simulink model "SUPERSONIC_ALTITUDEHOLD_AUTOPILOT_SIMULINK"  (R2020a)
settings: Solver=VariableStepAuto  StartTime=0.0  StopTime=150  RelTol=1e-3
values from neighbouring files (symbols this model uses):
  u0 = 1742    [SUPERSONIC_ALTITUDEHOLD_AUTOPILOT_MATLAB.m]
libraries: cstblocks x3, simulink x1
settings Model: Creator=AHSAN  LastModifiedBy=AHSAN

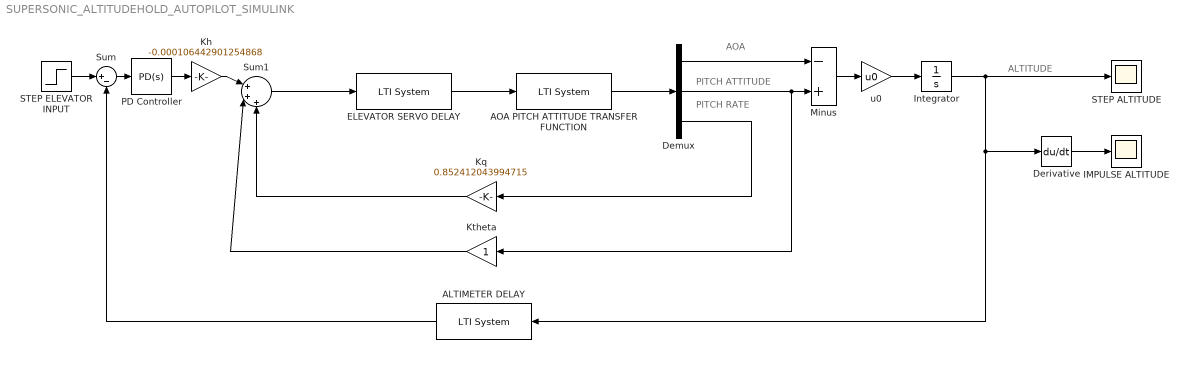
== system SUPERSONIC_ALTITUDEHOLD_AUTOPILOT_SIMULINK ==
  note: ALTITUDE
  note: PITCH RATE
  note: PITCH ATTITUDE
  note: AOA
  ALTIMETER DELAY : cstblocks/LTI System  sys=tf(1,[1 1])  IC=[]
  AOA PITCH ATTITUDE TRANSFER FUNCTION : cstblocks/LTI System  sys=SYSTEM  IC=[]
  Demux : Demux  Outputs=3
  Derivative : Derivative
  ELEVATOR SERVO DELAY : cstblocks/LTI System  sys=tf(10,[1 10])  IC=[]
  IMPULSE ALTITUDE : Scope
  Integrator : Integrator
  Kh : Gain  Gain=-0.000106442901254868
  Kq : Gain  Gain=0.852412043994715
  Ktheta : Gain
  Minus : Sum  Inputs=-+
  PD Controller : simulink/Continuous/PID Controller  Controller=PD  Form=Parallel  TimeDomain=Continuous-time  UseExternalTs=off  SampleTime=-1  IntegratorMethod=Forward Euler  FilterMethod=Forward Euler  ControllerParametersSource=internal  P=0.702446637657272  I=0  D=2.92686099023863  UseFilter=on  N=100  TunerSelectOption=Transfer Function Based (PID Tuner App)  InitialConditionSource=internal  InitialConditionForIntegrator=0  InitialConditionForFilter=0  DifferentiatorICPrevScaledInput=0  ExternalReset=none  TrackingMode=off  Kt=1  LimitOutput=off  UpperSaturationLimit=inf  LowerSaturationLimit=-inf  LinearizeAsGain=on  AntiWindupMode=none  Kb=1  POutMin=[]  POutMax=[]  IOutMin=[]  IOutMax=[]  DOutMin=[]  DOutMax=[]  NOutMin=[]  NOutMax=[]  SumOutMin=[]  SumOutMax=[]  SaturationOutMin=[]  SaturationOutMax=[]  PParamMin=[]  PParamMax=[]  IParamMin=[]  IParamMax=[]  DParamMin=[]  DParamMax=[]  NParamMin=[]  NParamMax=[]  KbParamMin=[]  KbParamMax=[]  KtParamMin=[]  KtParamMax=[]  KbOutMin=[]  KbOutMax=[]  KtOutMin=[]  KtOutMax=[]  IntegratorOutMin=[]  IntegratorOutMax=[]  FilterOutMin=[]  FilterOutMax=[]  SumI1OutMin=[]  SumI1OutMax=[]  SumI2OutMin=[]  SumI2OutMax=[]  SumI3OutMin=[]  SumI3OutMax=[]  SumI4OutMin=[]  SumI4OutMax=[]  SumDOutMin=[]  SumDOutMax=[]  DifferentiatorOutMin=[]  DifferentiatorOutMax=[]  FilterDiffOutCoefMin=[]  FilterDiffOutCoefMax=[]  ReciprocalOutMin=[]  ReciprocalOutMax=[]  SumDenOutMin=[]  SumDenOutMax=[]  SumNumOutMin=[]  SumNumOutMax=[]  DivideOutMin=[]  DivideOutMax=[]  UdiffTsProdOutMin=[]  UdiffTsProdOutMax=[]  NTsProdOutMin=[]  NTsProdOutMax=[]  UintegralTsProdOutMin=[]  UintegralTsProdOutMax=[]  UngainTsProdOutMin=[]  UngainTsProdOutMax=[]  IntegratorContinuousStateAttributes=''  IntegratorStateMustResolveToSignalObject=off  IntegratorRTWStateStorageClass=Auto  FilterContinuousStateAttributes=''  FilterStateMustResolveToSignalObject=off  FilterRTWStateStorageClass=Auto  ParallelPVariant=InternalParameters  IdealPVariant=Disabled  IVariant=Disabled  DVariant=InternalParameters  IntegratorVariant=Disabled  SatVariant=Disabled  AWVariant=Disabled  PCopyVariant=Disabled  TRVariant=Disabled  FdbkBlocksVariant=Forward  IdealPFdbkVariant=Disabled  SatFdbkVariant=Disabled  DerivativeFilterVariant=ContFilter  NVariant=InternalParameters  NCopyVariant=Disabled  FilterICVariant=InternalICsFilter  IntegratorICVariant=Disabled  ExternalResetVariant=Disabled  TRSumVariant=Passthrough  SumFdbkVariant=Disabled  SumVariant=Sum_PD  TsampFilterVariant=InternalTs  TsampNgainVariant=Passthrough  TsampIntegralVariant=Disabled_SignalSpec
  STEP ALTITUDE : Scope
  STEP ELEVATOR INPUT : Step  Time=0  SampleTime=0
  Sum : Sum  Inputs=|+-
  Sum1 : Sum  Inputs=|+++
  u0 : Gain  Gain=u0
  wires:
  ELEVATOR SERVO DELAY/1 -> AOA PITCH ATTITUDE TRANSFER FUNCTION/1
  AOA PITCH ATTITUDE TRANSFER FUNCTION/1 -> Demux/1
  Minus/1 -> u0/1
  u0/1 -> Integrator/1
  Integrator/1 -> STEP ALTITUDE/1, Derivative/1, ALTIMETER DELAY/1
  STEP ELEVATOR INPUT/1 -> Sum/1
  ALTIMETER DELAY/1 -> Sum/2
  Kh/1 -> Sum1/1
  Demux/2 -> Minus/2, Ktheta/1
  Demux/1 -> Minus/1
  Sum1/1 -> ELEVATOR SERVO DELAY/1
  Demux/3 -> Kq/1
  Kq/1 -> Sum1/3
  Ktheta/1 -> Sum1/2
  Sum/1 -> PD Controller/1
  PD Controller/1 -> Kh/1
  Derivative/1 -> IMPULSE ALTITUDE/1
